simulink model "Maglev_SMC_block_test"  (R2025a)
settings: Solver=ode15s  StartTime=0.0  StopTime=T_sim  FixedStep=0.001  RelTol=1e-3
PreLoadFcn:
  | % Modellpfad abrufen
  | modelPath = fileparts(which(bdroot));
  | projectRoot = fileparts(modelPath);
  | 
  | % Simulationsumgebung einrichten und Parameter laden
  | run(fullfile(projectRoot, 'setup_sim_params.m'));
  | load(fullfile(projectRoot, 'Controller_Params', 'EKFData.mat'));
  | load(fullfile(projectRoot, 'Controller_Params', 'NonlinearControllerData.mat'));
undefined symbols (not defined in the file): airgap_eq, Ext_Fina_Val, Ext_Init_Val, grav, I_max, I_min, Km, mass, T_stp
libraries: fl_lib x11, nesl_utility x4, slctrl_smc x1
settings Model: Creator=Polarstern  LastModifiedBy=CelestialAurora
settings DebuggingCC: AlgebraicLoopMsg=none

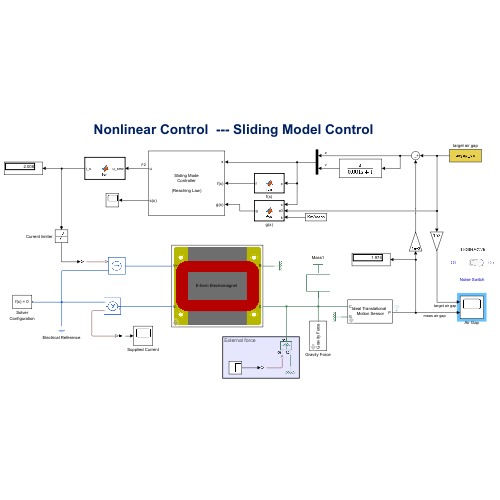
[thumbnail: Simulink's stored preview of the top-level diagram]
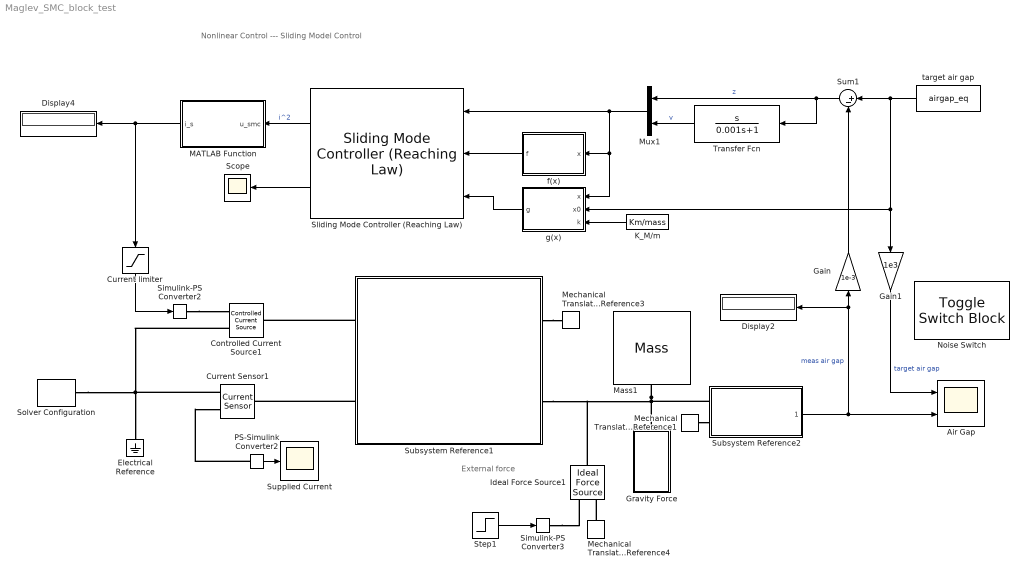
== system Maglev_SMC_block_test ==
  note: External force
  note: Nonlinear Control --- Sliding Model Control
  Air Gap : Scope  NumInputPorts=2
      settings: Title=Air Gap  ActiveDisplayYMinimum=0.88792767969619657  ActiveDisplayYMaximum=3.5819046117423423  DataLoggingVariableName=ScopeData4
  Controlled Current Source1 : fl_lib/Electrical/Electrical Sources/Controlled Current Source
  Current Sensor1 : fl_lib/Electrical/Electrical Sensors/Current Sensor
  Current limiter : Saturate  UpperLimit=I_max  LowerLimit=I_min
  Display2 : Display
  Display4 : Display
  Electrical Reference : fl_lib/Electrical/Electrical Elements/Electrical Reference
  Gain : Gain  Gain=1e-3
  Gain1 : Gain  Gain=1e3
  Gravity Force : Subsystem
      mask DialogControl DescGroupVar Prompt: Gravity Force
      mask DialogControl DescTextVar Prompt: Fg = Mass*grav, as constant parameters predefined
      mask DialogControl DescTextVar2 Prompt: Direction: Downward
      mask Display: disp("Gravity Force")
  Ideal Force Source1 : fl_lib/Mechanical/Mechanical Sources/Ideal Force Source
  K_M/m : Constant  Value=Km/mass
  MATLAB Function : MATLAB Function  TreatAsAtomicUnit=on
  Mass1 : fl_lib/Mechanical/Translational Elements/Mass  mass=mass kg  num_ports=foundation.enum.numPorts2.one  v_specify=on  v_priority=Low  v=0 m/s  v_nominal_specify=off  v_nominal_value=1  v_nominal_unit=m/s  f_specify=off  f_priority=None  f=0 N  f_nominal_specify=off  f_nominal_value=700  f_nominal_unit=N
  Mechanical Translational Reference1 : fl_lib/Mechanical/Translational Elements/Mechanical Translational Reference
  Mechanical Translational Reference3 : fl_lib/Mechanical/Translational Elements/Mechanical Translational Reference
  Mechanical Translational Reference4 : fl_lib/Mechanical/Translational Elements/Mechanical Translational Reference
  Mux1 : Mux  Inputs=2
  Noise Switch : ToggleSwitchBlock
  PS-Simulink Converter2 : nesl_utility/PS-Simulink Converter  PhysicalDomain=network_engine_domain  SubClassName=ps_output  LeftPortType=input  RightPortType=output  PseudoPeriodic=off  Frequencies=[]  VectorFormat=inherit  Unit=inherit  AffineConversion=off
  Scope : Scope
      settings: ActiveDisplayYMinimum=-0.395937143803728  ActiveDisplayYMaximum=0.088437460422636435
  Simulink-PS Converter2 : nesl_utility/Simulink-PS Converter  PhysicalDomain=network_engine_domain  SubClassName=ps_input  LeftPortType=input  RightPortType=output  PseudoPeriodic=off  Frequencies=[]  NoiseDistribution=none  NoiseParameters=[]  Unit=1  AffineConversion=off  FilteringAndDerivatives=zero  SimscapeFilterOrder=1  InputFilterTimeConstant=0.001  UdotUserProvided=0
  Simulink-PS Converter3 : nesl_utility/Simulink-PS Converter  PhysicalDomain=network_engine_domain  SubClassName=ps_input  LeftPortType=input  RightPortType=output  PseudoPeriodic=off  Frequencies=[]  NoiseDistribution=none  NoiseParameters=[]  Unit=1  AffineConversion=off  FilteringAndDerivatives=provide  SimscapeFilterOrder=1  InputFilterTimeConstant=0.001  UdotUserProvided=0
  Sliding Mode Controller (Reaching Law) : slctrl_smc/Sliding Mode Controller (Reaching Law)  TaskMode=Regulation Mode  SlidingMatrix=smc.C  EnableTrackingDerivative=off  EnableSwitchingFunction=on  ReachingLaw=Exponential  ReachingRate=smc.eta  ControlGain=smc.K  PowerRate=0.01  BoundaryLayer=Saturation  Phi=smc.phi
  Solver Configuration : nesl_utility/Solver Configuration  PhysicalDomain=network_engine_domain  SubClassName=solver  LeftPortType=input  RightPortType=generic  Tones=[]  Harmonics=[]  SimulateNoise=off  Profile=off  UseLocalSampling=off  EnableSwitchedLinearOptims=on  FrequencyDomain=off  UseCCode=off  RelTol=0.001  AbsTol=1e-06  MinStep=1e-09  ToWorkspace=off  RevertToSquareIcSolve=off  NumHomotopyIterations=100  PhasorMode=off  PhasorModeNumHarmonics=1  ConsistencySolver=NEWTON_XTOL_AFTER_FTOL  IndexReductionMethod=DerivativeReplacement  DoDC=off  ResidualTolerance=1e-09  ConsistencyTolSource=GLOBAL  ConsistencyAbsTol=0.001  ConsistencyRelTol=0.001  ConsistencyTolFactor=0.001  UseLocalSolver=off  LocalSolverChoice=NE_BACKWARD_EULER_ADVANCER  ResolveIndetEquations=on  FunctionEvalNumThread=1  LocalSolverSampleTime=0.001  DoFixedCost=off  MaxNonlinIter=3  MaxModeIter=2  ComputeImpulses=off  ImpulseIterations=2  LinearAlgebra=auto  LinearAlgebraNumThread=0  EquationFormulation=NE_TIME_EF  DelaysMemoryBudget=1024  AutomaticFiltering=on  FilteringTimeConstant=0.001  PartitionStorageMethod=AS_NEEDED  PartitionMemoryBudget=1024  PartitionMethod=ROBUST  MultibodyUseLocalSolver=off  MultibodyLocalSolverChoice=ODE1  MultibodyLocalSolverSampleTime=0.001
  Step1 : Step  Time=T_stp  Before=Ext_Init_Val  After=Ext_Fina_Val  SampleTime=0
  Subsystem Reference1 : Subsystem  ReferencedSubsystem=IntegratedElectromagnet  l_airgap=airgap_init
  Subsystem Reference2 : Subsystem  ReferencedSubsystem=IdealTrans_MotionSensor  ns_sw=isNoiseActive  ns_pw=NoisePower  ts=Ts  init_pos=airgap_init
  Sum1 : Sum  Inputs=|+-
  Supplied Current : Scope
      settings: ActiveDisplayYMinimum=-1.7133540055206153  ActiveDisplayYMaximum=15.420186049685542  DataLoggingVariableName=ScopeData5
  Transfer Fcn : TransferFcn  Numerator=[1 0]  Denominator=[0.001 1]
  f(x) : MATLAB Function  TreatAsAtomicUnit=on
  g(x) : MATLAB Function  TreatAsAtomicUnit=on
  target air gap : Constant  Value=airgap_eq
  wires:
  f(x)/1(f) -> Sliding Mode Controller (Reaching Law)/2
  g(x)/1(g) -> Sliding Mode Controller (Reaching Law)/3
  Sliding Mode Controller (Reaching Law)/2 -> Scope/1
  Sliding Mode Controller (Reaching Law)/1 -> MATLAB Function/1(u_smc)  "i^2"
  K_M/m/1 -> g(x)/3(k)
  Sum1/1 -> Transfer Fcn/1, Mux1/1  "z"
  Current limiter/1 -> Simulink-PS Converter2/1
  Step1/1 -> Simulink-PS Converter3/1
  Transfer Fcn/1 -> Mux1/2  "v"
  MATLAB Function/1(i_s) -> Display4/1, Current limiter/1
  target air gap/1 -> Sum1/1, g(x)/2(x0), Gain1/1
  PS-Simulink Converter2/1 -> Supplied Current/1
  Mux1/1 -> g(x)/1(x), f(x)/1(x), Sliding Mode Controller (Reaching Law)/1
  Subsystem Reference2/1 -> Gain/1, Display2/1, Air Gap/2  "meas air gap"
  Gain/1 -> Sum1/2
  Gain1/1 -> Air Gap/1  "target air gap"
  connections:
  Mass1/LConn1 -- Subsystem Reference2/LConn1 -- Gravity Force/RConn1 -- Ideal Force Source1/LConn1 -- Subsystem Reference1/RConn2
  Controlled Current Source1/RConn2 -- Current Sensor1/RConn2 -- Electrical Reference/LConn1 -- Solver Configuration/RConn1
  Mechanical Translational Reference4/LConn1 -- Ideal Force Source1/RConn2
  PS-Simulink Converter2/LConn1 -- Current Sensor1/RConn1
  Simulink-PS Converter2/RConn1 -- Controlled Current Source1/RConn1
  Subsystem Reference1/LConn1 -- Controlled Current Source1/LConn1
  Simulink-PS Converter3/RConn1 -- Ideal Force Source1/RConn1
  Subsystem Reference1/RConn1 -- Mechanical Translational Reference3/LConn1
  Subsystem Reference1/LConn2 -- Current Sensor1/LConn1
  Mechanical Translational Reference1/LConn1 -- Subsystem Reference2/LConn2

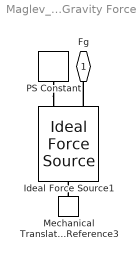
== system Maglev_SMC_block_test/Gravity Force ==
  Ideal Force Source1 : fl_lib/Mechanical/Mechanical Sources/Ideal Force Source
  Mechanical Translational Reference3 : fl_lib/Mechanical/Translational Elements/Mechanical Translational Reference
  PS Constant : fl_lib/Physical Signals/Sources/PS Constant  constant=mass*grav N
  Fg : PMIOPort  Side=Right
  connections:
  Mechanical Translational Reference3/LConn1 -- Ideal Force Source1/LConn1
  PS Constant/RConn1 -- Ideal Force Source1/RConn1
  Ideal Force Source1/RConn2 -- Fg/RConn1

== matlab function Maglev_SMC_block_test/f(x) ==
  data: x input; f output
function f = fcn(x)
    g_grav = 9.81;  % Gravity constant
    f = [x(2); -g_grav];

== matlab function Maglev_SMC_block_test/MATLAB Function ==
  data: u_smc input; i_s output
function i_s = fcn(u_smc)
% Recover actual current from u = i_s^2
i_s = sqrt(max(u_smc, 0));

== matlab function Maglev_SMC_block_test/g(x) ==
  data: x input; g output; x0 input; k input
function g = fcn(x, x0, k)
    
% x  = [x1; x2]
    % x0 = equilibrium air gap
    % k  = Km/m
    x_gap = x0 - x(1);
    x_gap = max(x_gap, 1e-5);      % singularity protection
    g = [0; k / x_gap^2];         % [0; (Km/m)/(x0-x1)^2]
